simulink model "gm_sampleModel1395_sub"  (R2023a)
settings: Solver=VariableStepAuto  StartTime=0.0  StopTime=10.0  RelTol=1e-3
libraries: simulink x1
settings Model: Creator=user1  LastModifiedBy=user1
settings OptimizationCC: BlockReduction=off  ConditionallyExecuteInputs=off
settings DebuggingCC: InheritedTsInSrcMsg=none

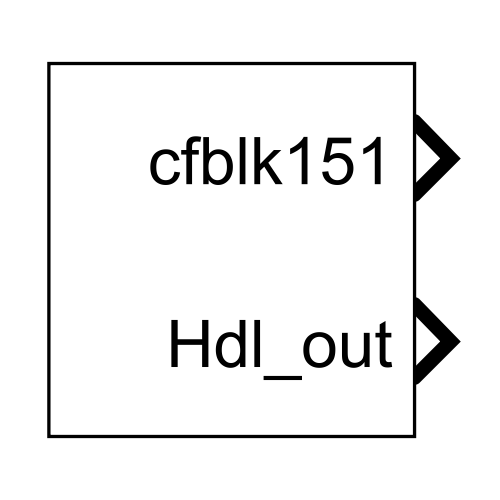
[thumbnail: Simulink's stored preview of the top-level diagram]
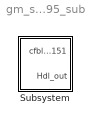
== system gm_sampleModel1395_sub ==
  Subsystem : Subsystem

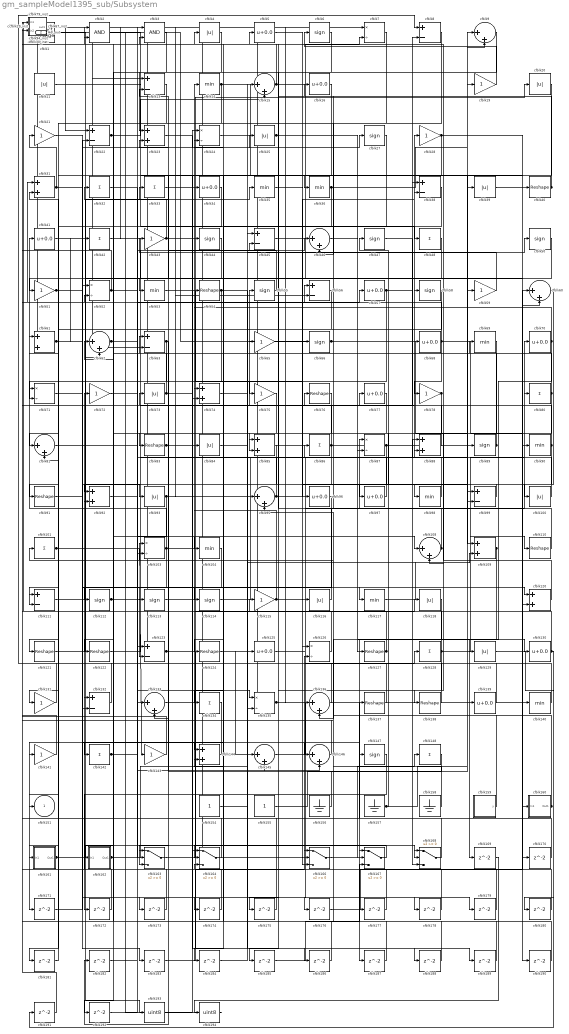
== system gm_sampleModel1395_sub/Subsystem ==
  cfblk1 : simulink/Logic and Bit Operations/Detect Change  vinit=0  OutDataTypeStr=uint8
      settings: LibrarySourceBlock=|
      | hdlsllib/Logic and Bit
      | Operations/Detect
      | Change
  cfblk{4,11,20,25,39,73,84,93,100,116,118,129} (12 alike) : Abs  OutDataTypeStr=uint8  SaturateOnIntegerOverflow=off
  cfblk{32..33,42,48,80,86,101,128,134,142,148} (11 alike) : Sum  Inputs=+  OutDataTypeStr=uint8
  cfblk{7,24,52,71,87,103,126,135} (8 alike) : Product  Inputs=*/  OutDataTypeStr=uint8  RndMeth=Zero  SaturateOnIntegerOverflow=on
  cfblk{14,35..36,53,69,90,98,104,117,140} (10 alike) : MinMax  OutDataTypeStr=uint8
  cfblk105_inst : Subsystem
  cfblk106_inst : Subsystem
  cfblk{9,15,46,60,62,81,95,108,133,136,145..146} (12 alike) : Sum  Inputs=|++  OutDataTypeStr=uint8
  cfblk{23,31,61,74,85,88,92,109,120,144} (10 alike) : Sum  OutDataTypeStr=uint8
  cfblk{40,54,76,83,91,110,121..122,124,127,137..138} (12 alike) : Reshape
  cfblk{8,13,22,38,45,56,63,99,111,123,132} (11 alike) : Sum  Inputs=+-  OutDataTypeStr=uint8
  cfblk{6,27,44,47,50,55,58,66,89,112..114,147} (13 alike) : Signum
  cfblk{19,21,28,43,51,59,65,72,75,78,115,131,141,143} (14 alike) : Gain  OutDataTypeStr=uint8
  cfblk119_inst : Subsystem
  cfblk{5,16,34,41,57,68,70,77,96..97,125,130,139} (13 alike) : Bias  Bias=0.0  SaturateOnIntegerOverflow=off
  cfblk12_inst : Subsystem
  cfblk154 : Constant  OutDataTypeStr=uint8  SampleTime=-1
  cfblk155 : Constant  OutDataTypeStr=uint8  SampleTime=-1
  cfblk156 : Ground
  cfblk157 : Ground
  cfblk158 : Ground
  cfblk159 : Subsystem  mask(Counter Free-Running){NumBits=double(16), tsamp=double(-1)}
      mask prompts: NumBits "Simulink:masks:NumberOfBits_MP"; tsamp "Simulink:masks:SampleTime_MP"
      mask help: Simulink:masks:CounterFreeRunning_MD
  cfblk160 : Subsystem
  cfblk161 : Subsystem
  cfblk162 : Subsystem
  cfblk{163..164,166..168} (5 alike) : Switch  OutDataTypeStr=uint8  SaturateOnIntegerOverflow=off  InputSameDT=off
  cfblk{169..192} (24 alike) : Delay  SampleTime=1
  cfblk17_inst : Subsystem
  cfblk18_inst : Subsystem
  cfblk193 : DataTypeConversion  OutDataTypeStr=uint8  SaturateOnIntegerOverflow=off  RndMeth=Floor
  cfblk194 : DataTypeConversion  OutDataTypeStr=uint8  SaturateOnIntegerOverflow=off  RndMeth=Floor
  cfblk2 : Logic  AllPortsSameDT=off  OutDataTypeStr=boolean
  cfblk29_inst : Subsystem
  cfblk3 : Logic  AllPortsSameDT=off  OutDataTypeStr=boolean
  cfblk30_inst : Subsystem
  cfblk64_inst : Subsystem
  cfblk67_inst : Subsystem
  cfblk79_inst : Subsystem
  cfblk94_inst : Subsystem
  cfblk151 : Outport  OutDataTypeStr=uint8  VectorParamsAs1DForOutWhenUnconnected=off
  Hdl_out : Outport  Port=2  OutDataTypeStr=uint8  SampleTime=1
  wires:
  cfblk1/1 -> cfblk193/1
  cfblk100/1 -> cfblk28/1
  cfblk101/1 -> cfblk45/2, cfblk143/1
  cfblk103/1 -> cfblk41/1, cfblk123/2, cfblk86/1
  cfblk104/1 -> cfblk182/1
  cfblk105_inst/1(out1) -> cfblk140/1
  cfblk106_inst/1(out1) -> cfblk89/1
  cfblk108/1 -> cfblk73/1, cfblk87/1
  cfblk109/1 -> cfblk136/2, cfblk169/1
  cfblk11/1 -> cfblk48/1
  cfblk110/1 -> cfblk56/1
  cfblk111/1 -> cfblk35/1
  cfblk112/1 -> cfblk88/2, cfblk117/1
  cfblk113/1 -> cfblk45/1
  cfblk114/1 -> cfblk88/1
  cfblk115/1 -> cfblk9/1, cfblk14/1
  cfblk116/1 -> cfblk119_inst/1(in1)
  cfblk117/1 -> cfblk110/1
  cfblk118/1 -> cfblk187/1
  cfblk119_inst/1(out1) -> cfblk96/1, cfblk56/2
  cfblk12_inst/1(out1) -> cfblk139/1
  cfblk120/1 -> cfblk67_inst/1(in1)
  cfblk121/1 -> cfblk62/2
  cfblk122/1 -> cfblk58/1
  cfblk123/1 -> cfblk118/1, cfblk188/1
  cfblk124/1 -> cfblk145/1
  cfblk125/1 -> cfblk70/1
  cfblk126/1 -> cfblk33/1
  cfblk127/1 -> cfblk81/2, cfblk72/1
  cfblk128/1 -> cfblk30_inst/1(in1), cfblk185/1, cfblk80/1
  cfblk129/1 -> cfblk191/1
  cfblk13/1 -> cfblk71/2
  cfblk130/1 -> cfblk30_inst/2(in2), cfblk180/1
  cfblk131/1 -> cfblk8/1
  cfblk132/1 -> cfblk79_inst/2(in2)
  cfblk133/1 -> cfblk20/1
  cfblk134/1 -> cfblk171/1
  cfblk135/1 -> cfblk59/1, cfblk179/1
  cfblk136/1 -> cfblk94_inst/1(in1)
  cfblk137/1 -> cfblk106_inst/1(in1)
  cfblk138/1 -> cfblk32/1
  cfblk139/1 -> cfblk18_inst/1(in1)
  cfblk14/1 -> cfblk99/1, cfblk81/1, cfblk151/1
  cfblk140/1 -> cfblk123/1
  cfblk141/1 -> cfblk119_inst/2(in2)
  cfblk142/1 -> cfblk146/2, cfblk192/1
  cfblk143/1 -> cfblk12_inst/1(in1)
  cfblk144/1 -> cfblk141/1
  cfblk145/1 -> cfblk128/1
  cfblk146/1 -> cfblk12_inst/2(in2)
  cfblk147/1 -> cfblk172/1
  cfblk148/1 -> cfblk145/2
  cfblk15/1 -> cfblk67_inst/2(in2), cfblk168/3, cfblk7/2, cfblk90/1
  cfblk154/1 -> cfblk15/1
  cfblk155/1 -> cfblk39/1
  cfblk156/1 -> cfblk63/1
  cfblk157/1 -> cfblk47/1, cfblk19/1
  cfblk158/1 -> cfblk115/1
  cfblk159/1(y) -> cfblk103/1
  cfblk16/1 -> cfblk111/2
  cfblk160/1(Out1) -> cfblk95/2, cfblk101/1
  cfblk161/1(Out1) -> cfblk167/1, cfblk176/1
  cfblk162/1(Out1) -> cfblk74/1, cfblk50/1
  cfblk163/1 -> cfblk55/1
  cfblk164/1 -> cfblk92/2
  cfblk166/1 -> cfblk148/1
  cfblk167/1 -> cfblk164/2
  cfblk168/1 -> cfblk137/1
  cfblk169/1 -> cfblk194/1
  cfblk17_inst/1(out1) -> cfblk44/1
  cfblk170/1 -> cfblk24/2
  cfblk171/1 -> cfblk22/2
  cfblk172/1 -> cfblk29_inst/1(in1)
  cfblk173/1 -> cfblk132/1
  cfblk174/1 -> cfblk52/2
  cfblk175/1 -> cfblk79_inst/1(in1)
  cfblk176/1 -> cfblk60/1
  cfblk177/1 -> cfblk126/2
  cfblk178/1 -> cfblk17_inst/2(in2)
  cfblk179/1 -> cfblk61/1
  cfblk18_inst/1(out1) -> cfblk63/2
  cfblk180/1 -> cfblk164/3
  cfblk181/1 -> cfblk31/2
  cfblk182/1 -> cfblk133/1
  cfblk183/1 -> cfblk166/1
  cfblk184/1 -> cfblk109/2
  cfblk185/1 -> cfblk167/3
  cfblk186/1 -> cfblk64_inst/2(in2)
  cfblk187/1 -> cfblk62/1
  cfblk188/1 -> cfblk144/2
  cfblk189/1 -> cfblk164/1
  cfblk19/1 -> cfblk6/1
  cfblk190/1 -> cfblk136/1
  cfblk191/1 -> cfblk94_inst/2(in2)
  cfblk192/1 -> cfblk27/1
  cfblk193/1 -> cfblk34/1
  cfblk194/1 -> cfblk1/1
  cfblk2/1 -> cfblk74/2
  cfblk20/1 -> cfblk144/1
  cfblk21/1 -> cfblk52/1
  cfblk22/1 -> cfblk15/2, cfblk170/1
  cfblk23/1 -> cfblk146/1
  cfblk24/1 -> cfblk66/1
  cfblk25/1 -> cfblk166/2, cfblk130/1
  cfblk27/1 -> cfblk75/1
  cfblk28/1 -> cfblk190/1, cfblk53/1
  cfblk29_inst/1(out1) -> cfblk125/1
  cfblk3/1 -> cfblk23/1
  cfblk30_inst/1(out1) -> cfblk11/1
  cfblk31/1 -> cfblk120/1, cfblk21/1
  cfblk32/1 -> cfblk104/1
  cfblk33/1 -> cfblk36/1
  cfblk34/1 -> cfblk51/1
  cfblk35/1 -> cfblk98/1
  cfblk36/1 -> cfblk9/2, cfblk175/1
  cfblk38/1 -> cfblk184/1
  cfblk39/1 -> cfblk40/1
  cfblk4/1 -> cfblk122/1
  cfblk40/1 -> cfblk5/1, cfblk3/2
  cfblk41/1 -> cfblk160/1(In1)
  cfblk42/1 -> cfblk60/2
  cfblk43/1 -> cfblk2/1, cfblk178/1
  cfblk44/1 -> cfblk161/1(In1)
  cfblk45/1 -> cfblk127/1
  cfblk46/1 -> cfblk87/2
  cfblk47/1 -> cfblk99/2
  cfblk48/1 -> cfblk181/1
  cfblk5/1 -> cfblk116/1
  cfblk50/1 -> cfblk166/3
  cfblk51/1 -> cfblk93/1, cfblk24/1
  cfblk52/1 -> cfblk64_inst/1(in1), cfblk46/1
  cfblk53/1 -> cfblk126/1
  cfblk54/1 -> cfblk168/2, cfblk133/2
  cfblk55/1 -> cfblk13/2
  cfblk56/1 -> cfblk121/1
  cfblk57/1 -> cfblk8/2, cfblk163/3, cfblk131/1
  cfblk58/1 -> cfblk71/1
  cfblk59/1 -> cfblk43/1
  cfblk6/1 -> cfblk85/2
  cfblk60/1 -> cfblk100/1
  cfblk61/1 -> cfblk174/1, cfblk173/1, cfblk42/1
  cfblk62/1 -> cfblk57/1, cfblk114/1
  cfblk63/1 -> cfblk91/1, cfblk83/1
  cfblk64_inst/1(out1) -> cfblk61/2, cfblk167/2, cfblk13/1
  cfblk65/1 -> cfblk168/1
  cfblk66/1 -> cfblk109/1, Hdl_out/1
  cfblk67_inst/1(out1) -> cfblk7/1
  cfblk68/1 -> cfblk31/1, cfblk120/2, cfblk105_inst/1(in1), cfblk78/1
  cfblk69/1 -> cfblk138/1
  cfblk7/1 -> cfblk46/2
  cfblk70/1 -> cfblk54/1, cfblk4/1, cfblk129/1
  cfblk71/1 -> cfblk147/1
  cfblk72/1 -> cfblk25/1
  cfblk73/1 -> cfblk18_inst/2(in2), cfblk189/1
  cfblk74/1 -> cfblk177/1
  cfblk75/1 -> cfblk142/1
  cfblk76/1 -> cfblk163/1
  cfblk77/1 -> cfblk85/1
  cfblk78/1 -> cfblk163/2, cfblk124/1
  cfblk79_inst/1(out1) -> cfblk22/1
  cfblk8/1 -> cfblk111/1
  cfblk80/1 -> cfblk97/1, cfblk69/1
  cfblk81/1 -> cfblk135/1
  cfblk83/1 -> cfblk76/1, cfblk38/1
  cfblk84/1 -> cfblk186/1
  cfblk85/1 -> cfblk134/1
  cfblk86/1 -> cfblk23/2, cfblk113/1
  cfblk87/1 -> cfblk135/2, cfblk103/2
  cfblk88/1 -> cfblk17_inst/1(in1)
  cfblk89/1 -> cfblk68/1, cfblk2/2, cfblk105_inst/2(in2)
  cfblk9/1 -> cfblk112/1
  cfblk90/1 -> cfblk77/1, cfblk108/2, cfblk65/1
  cfblk91/1 -> cfblk183/1
  cfblk92/1 -> cfblk108/1
  cfblk93/1 -> cfblk95/1, cfblk162/1(In1)
  cfblk94_inst/1(out1) -> cfblk29_inst/2(in2), cfblk106_inst/2(in2)
  cfblk95/1 -> cfblk84/1, cfblk38/2
  cfblk96/1 -> cfblk132/2
  cfblk97/1 -> cfblk16/1
  cfblk98/1 -> cfblk3/1
  cfblk99/1 -> cfblk92/1

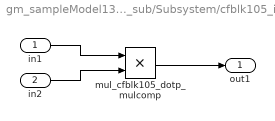
== system gm_sampleModel1395_sub/Subsystem/cfblk105_inst ==
  in1 : Inport  OutDataTypeStr=uint8  SampleTime=1
  in2 : Inport  Port=2  OutDataTypeStr=uint8  SampleTime=1
  mul_cfblk105_dotp_mulcomp : Product  Inputs=**  OutDataTypeStr=uint8  SampleTime=1
  out1 : Outport  OutDataTypeStr=uint8  SampleTime=1
  wires:
  in1/1 -> mul_cfblk105_dotp_mulcomp/1
  in2/1 -> mul_cfblk105_dotp_mulcomp/2
  mul_cfblk105_dotp_mulcomp/1 -> out1/1

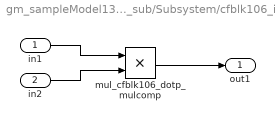
== system gm_sampleModel1395_sub/Subsystem/cfblk106_inst ==
  in1 : Inport  OutDataTypeStr=uint8  SampleTime=1
  in2 : Inport  Port=2  OutDataTypeStr=uint8  SampleTime=1
  mul_cfblk106_dotp_mulcomp : Product  Inputs=**  OutDataTypeStr=uint8  SampleTime=1
  out1 : Outport  OutDataTypeStr=uint8  SampleTime=1
  wires:
  in1/1 -> mul_cfblk106_dotp_mulcomp/1
  in2/1 -> mul_cfblk106_dotp_mulcomp/2
  mul_cfblk106_dotp_mulcomp/1 -> out1/1

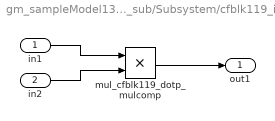
== system gm_sampleModel1395_sub/Subsystem/cfblk119_inst ==
  in1 : Inport  OutDataTypeStr=uint8  SampleTime=1
  in2 : Inport  Port=2  OutDataTypeStr=uint8  SampleTime=1
  mul_cfblk119_dotp_mulcomp : Product  Inputs=**  OutDataTypeStr=uint8  SampleTime=1
  out1 : Outport  OutDataTypeStr=uint8  SampleTime=1
  wires:
  in1/1 -> mul_cfblk119_dotp_mulcomp/1
  in2/1 -> mul_cfblk119_dotp_mulcomp/2
  mul_cfblk119_dotp_mulcomp/1 -> out1/1

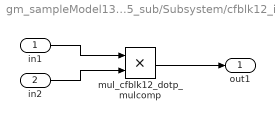
== system gm_sampleModel1395_sub/Subsystem/cfblk12_inst ==
  in1 : Inport  OutDataTypeStr=uint8  SampleTime=1
  in2 : Inport  Port=2  OutDataTypeStr=uint8  SampleTime=1
  mul_cfblk12_dotp_mulcomp : Product  Inputs=**  OutDataTypeStr=uint8  SampleTime=1
  out1 : Outport  OutDataTypeStr=uint8  SampleTime=1
  wires:
  in1/1 -> mul_cfblk12_dotp_mulcomp/1
  in2/1 -> mul_cfblk12_dotp_mulcomp/2
  mul_cfblk12_dotp_mulcomp/1 -> out1/1

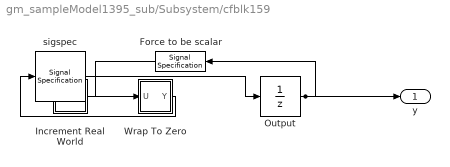
== system gm_sampleModel1395_sub/Subsystem/cfblk159 ==
  Force to be scalar : SignalSpecification  DisableCoverage=on  Dimensions=1
  Increment Real World : Subsystem  mask(Real World Value Increment){}
      mask help: Simulink:masks:RealWorldValueIncrement_MD
      mask Display: disp('V++')
  Output : UnitDelay  InitialCondition=0.0  SampleTime=tsamp  HasFrameUpgradeWarning=on
  Wrap To Zero : Subsystem  mask(Wrap To Zero){Threshold=double(65535)}
      mask prompts: Threshold "Simulink:masks:Threshold_MP"
      mask help: Simulink:masks:WrapToZero_MD
  sigspec : SignalSpecification  OutDataTypeStr=uint16  Dimensions=1
  y : Outport  SampleTime=1
  wires:
  Force to be scalar/1 -> Increment Real World/1(u)
  Increment Real World/1(y) -> Wrap To Zero/1(U)
  Output/1 -> Force to be scalar/1, y/1
  Wrap To Zero/1(Y) -> sigspec/1
  sigspec/1 -> Output/1

== system gm_sampleModel1395_sub/Subsystem/cfblk160 ==
  In1 : Inport  OutDataTypeStr=uint8  PortDimensions=1  SampleTime=1
  Out1 : Outport  SampleTime=1
  wires:
  In1/1 -> Out1/1

== system gm_sampleModel1395_sub/Subsystem/cfblk161 ==
  In1 : Inport  OutDataTypeStr=uint8  PortDimensions=1  SampleTime=1
  Out1 : Outport  SampleTime=1
  wires:
  In1/1 -> Out1/1

== system gm_sampleModel1395_sub/Subsystem/cfblk162 ==
  In1 : Inport  OutDataTypeStr=uint8  PortDimensions=1  SampleTime=1
  Out1 : Outport  SampleTime=1
  wires:
  In1/1 -> Out1/1

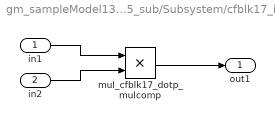
== system gm_sampleModel1395_sub/Subsystem/cfblk17_inst ==
  in1 : Inport  OutDataTypeStr=uint8  SampleTime=1
  in2 : Inport  Port=2  OutDataTypeStr=uint8  SampleTime=1
  mul_cfblk17_dotp_mulcomp : Product  Inputs=**  OutDataTypeStr=uint8  SampleTime=1
  out1 : Outport  OutDataTypeStr=uint8  SampleTime=1
  wires:
  in1/1 -> mul_cfblk17_dotp_mulcomp/1
  in2/1 -> mul_cfblk17_dotp_mulcomp/2
  mul_cfblk17_dotp_mulcomp/1 -> out1/1

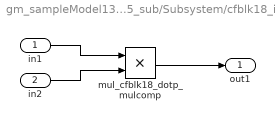
== system gm_sampleModel1395_sub/Subsystem/cfblk18_inst ==
  in1 : Inport  OutDataTypeStr=uint8  SampleTime=1
  in2 : Inport  Port=2  OutDataTypeStr=uint8  SampleTime=1
  mul_cfblk18_dotp_mulcomp : Product  Inputs=**  OutDataTypeStr=uint8  SampleTime=1
  out1 : Outport  OutDataTypeStr=uint8  SampleTime=1
  wires:
  in1/1 -> mul_cfblk18_dotp_mulcomp/1
  in2/1 -> mul_cfblk18_dotp_mulcomp/2
  mul_cfblk18_dotp_mulcomp/1 -> out1/1

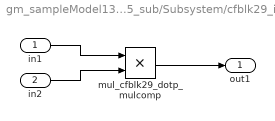
== system gm_sampleModel1395_sub/Subsystem/cfblk29_inst ==
  in1 : Inport  OutDataTypeStr=uint8  SampleTime=1
  in2 : Inport  Port=2  OutDataTypeStr=uint8  SampleTime=1
  mul_cfblk29_dotp_mulcomp : Product  Inputs=**  OutDataTypeStr=uint8  SampleTime=1
  out1 : Outport  OutDataTypeStr=uint8  SampleTime=1
  wires:
  in1/1 -> mul_cfblk29_dotp_mulcomp/1
  in2/1 -> mul_cfblk29_dotp_mulcomp/2
  mul_cfblk29_dotp_mulcomp/1 -> out1/1

== system gm_sampleModel1395_sub/Subsystem/cfblk30_inst ==
  in1 : Inport  OutDataTypeStr=uint8  SampleTime=1
  in2 : Inport  Port=2  OutDataTypeStr=uint8  SampleTime=1
  mul_cfblk30_dotp_mulcomp : Product  Inputs=**  OutDataTypeStr=uint8  SampleTime=1
  out1 : Outport  OutDataTypeStr=uint8  SampleTime=1
  wires:
  in1/1 -> mul_cfblk30_dotp_mulcomp/1
  in2/1 -> mul_cfblk30_dotp_mulcomp/2
  mul_cfblk30_dotp_mulcomp/1 -> out1/1

== system gm_sampleModel1395_sub/Subsystem/cfblk64_inst ==
  in1 : Inport  OutDataTypeStr=uint8  SampleTime=1
  in2 : Inport  Port=2  OutDataTypeStr=uint8  SampleTime=1
  mul_cfblk64_dotp_mulcomp : Product  Inputs=**  OutDataTypeStr=uint8  SampleTime=1
  out1 : Outport  OutDataTypeStr=uint8  SampleTime=1
  wires:
  in1/1 -> mul_cfblk64_dotp_mulcomp/1
  in2/1 -> mul_cfblk64_dotp_mulcomp/2
  mul_cfblk64_dotp_mulcomp/1 -> out1/1

== system gm_sampleModel1395_sub/Subsystem/cfblk67_inst ==
  in1 : Inport  OutDataTypeStr=uint8  SampleTime=1
  in2 : Inport  Port=2  OutDataTypeStr=uint8  SampleTime=1
  mul_cfblk67_dotp_mulcomp : Product  Inputs=**  OutDataTypeStr=uint8  SampleTime=1
  out1 : Outport  OutDataTypeStr=uint8  SampleTime=1
  wires:
  in1/1 -> mul_cfblk67_dotp_mulcomp/1
  in2/1 -> mul_cfblk67_dotp_mulcomp/2
  mul_cfblk67_dotp_mulcomp/1 -> out1/1

== system gm_sampleModel1395_sub/Subsystem/cfblk79_inst ==
  in1 : Inport  OutDataTypeStr=uint8  SampleTime=1
  in2 : Inport  Port=2  OutDataTypeStr=uint8  SampleTime=1
  mul_cfblk79_dotp_mulcomp : Product  Inputs=**  OutDataTypeStr=uint8  SampleTime=1
  out1 : Outport  OutDataTypeStr=uint8  SampleTime=1
  wires:
  in1/1 -> mul_cfblk79_dotp_mulcomp/1
  in2/1 -> mul_cfblk79_dotp_mulcomp/2
  mul_cfblk79_dotp_mulcomp/1 -> out1/1

== system gm_sampleModel1395_sub/Subsystem/cfblk94_inst ==
  in1 : Inport  OutDataTypeStr=uint8  SampleTime=1
  in2 : Inport  Port=2  OutDataTypeStr=uint8  SampleTime=1
  mul_cfblk94_dotp_mulcomp : Product  Inputs=**  OutDataTypeStr=uint8  SampleTime=1
  out1 : Outport  OutDataTypeStr=uint8  SampleTime=1
  wires:
  in1/1 -> mul_cfblk94_dotp_mulcomp/1
  in2/1 -> mul_cfblk94_dotp_mulcomp/2
  mul_cfblk94_dotp_mulcomp/1 -> out1/1

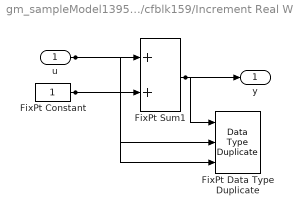
== system gm_sampleModel1395_sub/Subsystem/cfblk159/Increment Real World ==
  u : Inport  OutDataTypeStr=uint16  SampleTime=1
  FixPt Constant : Constant  DisableCoverage=on  OutDataTypeStr=Inherit: Inherit via back propagation  SampleTime=-1
  FixPt Data Type Duplicate : DataTypeDuplicate  DisableCoverage=on  NumInputPorts=3
  FixPt Sum1 : Sum  InputSameDT=on  OutDataTypeStr=Inherit: Inherit via back propagation  LockScale=on
  y : Outport  SampleTime=1
  wires:
  u/1 -> FixPt Sum1/1, FixPt Data Type Duplicate/2
  FixPt Constant/1 -> FixPt Sum1/2, FixPt Data Type Duplicate/3
  FixPt Sum1/1 -> FixPt Data Type Duplicate/1, y/1

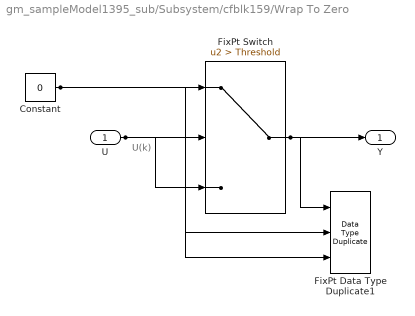
== system gm_sampleModel1395_sub/Subsystem/cfblk159/Wrap To Zero ==
  note: U(k)
  U : Inport  OutDataTypeStr=uint16  SampleTime=1
  Constant : Constant  DisableCoverage=on  Value=0  OutDataTypeStr=Inherit: Inherit via back propagation  SampleTime=-1
  FixPt Data Type Duplicate1 : DataTypeDuplicate  DisableCoverage=on  NumInputPorts=3
  FixPt Switch : Switch  Criteria=u2 > Threshold  Threshold=Threshold  OutDataTypeStr=Inherit: Inherit via back propagation  ZeroCross=off  SaturateOnIntegerOverflow=off  InputSameDT=off
  Y : Outport  SampleTime=1
  wires:
  U/1 -> FixPt Switch/3, FixPt Switch/2, FixPt Data Type Duplicate1/2
  Constant/1 -> FixPt Switch/1, FixPt Data Type Duplicate1/3
  FixPt Switch/1 -> FixPt Data Type Duplicate1/1, Y/1
